simulink library "myo_lib"  (R2019b)
settings: Solver=ode45  StartTime=0.0  StopTime=10.0  RelTol=1e-3  EnableMultiTasking=on
settings Model: Creator=Mark Tomaszewski  LastModifiedBy=bhisma
settings DataIOCC: LimitDataPoints=on  SaveFormat=Array  ReturnWorkspaceOutputs=off
settings OptimizationCC: LifeSpan=inf
settings DebuggingCC: UnderspecifiedInitializationDetection=Classic  MergeDetectMultiDrivingBlocksExec=none  SolverPrmCheckMsg=warning  StateNameClashWarn=warning  SFUnexpectedBacktrackingDiag=warning  SFNoUnconditionalDefaultTransitionDiag=warning  SFExecutionAtInitializationDiag=none  ArithmeticOperatorsInVariantConditions=warning
settings HardwareCC: ProdBitPerPointer=32  ProdBitPerSizeT=32  ProdBitPerPtrDiffT=32  ProdLargestAtomicFloat=None  ProdIntDivRoundTo=Undefined  ProdEndianess=Unspecified  ProdWordSize=32  ProdHWDeviceType=32-bit Generic
settings ModelReferenceCC: PropagateSignalLabelsOutOfModel=off
settings SFSimCC: SimUseLocalCustomCode=off  CustomCodeUndefinedFunction=UseInterfaceOnly
settings RTWCC: RTWUseLocalCustomCode=off
settings CodeAppCC: StateflowObjectComments=on
settings GRTTargetCC: TargetLangStandard=C89/C90 (ANSI)  GeneratePreprocessorConditionals=Disable all
settings ConfigComp: CovMetricSettings=dw  CovHtmlReporting=on  CovSaveCumulativeToWorkspaceVar=on  CovSaveSingleToWorkspaceVar=on  CovExternalEMLEnable=off

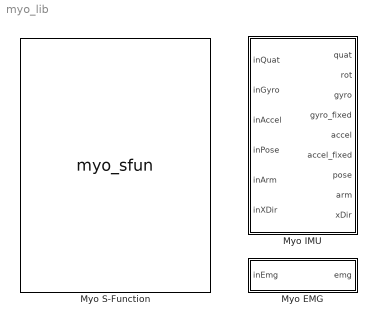
== system myo_lib ==
  Myo EMG : Subsystem
  Myo IMU : Subsystem
  Myo S-Function : S-Function  FunctionName=myo_sfun  Parameters=emgEnabled,countMyos  SFunctionDeploymentMode=off  EnableBusSupport=off  mask{emgEnabled=1, countMyos=1}
      mask prompts: emgEnabled "EMG Enabled (1 to set or 0 to unset)"; countMyos "Count Myos (1 or 2)"
      mask init:
      | disp init-mask
      mask Callback emgEnabled: myo_sfun_param_cb(gcb)
      mask Callback countMyos: myo_sfun_param_cb(gcb)
      mask Display:
      | %myo_sfun_draw_cb(gcb);
      | 
      | text(0.1,0.9,'Myo\nS-Function')
      | 
      | % default ports
      | port_label('output',1,'myoData(1).quat')
      | port_label('output',2,'myoData(1).gyro')
      | port_label('output',3,'myoData(1).accel')
      | port_label('output',4,'myoData(1).pose')
      | port_label('output',5,'myoData(1).arm')
      | port_label('output',6,'myoData(1).xDir')
      | 
      | % emg
      | if emgEnabled==1
      |   port_label('output',7,'myoData(1).emg')
      | end
      | 
      | % myo2
      | if countMyos==2
      |   port_label('output',7,'myoData(2).quat')
      |   port_label('output',8,'myoData(2).gyro')
      |   port_label('output',9,'myoData(2).accel')
      |   port_label('output',10,'myoData(2).pose')
      |   port_label('output',11,'myoData(2).arm')
      |   port_label('output',12,'myoData(2).xDir')
      | end

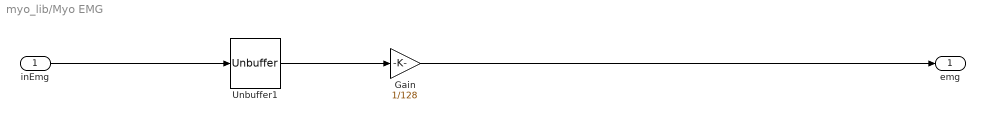
== system myo_lib/Myo EMG ==
  inEmg : Inport
  Gain : Gain  Gain=1/128
  Unbuffer1 : Unbuffer
  emg : Outport
  wires:
  Unbuffer1/1 -> Gain/1
  inEmg/1 -> Unbuffer1/1
  Gain/1 -> emg/1

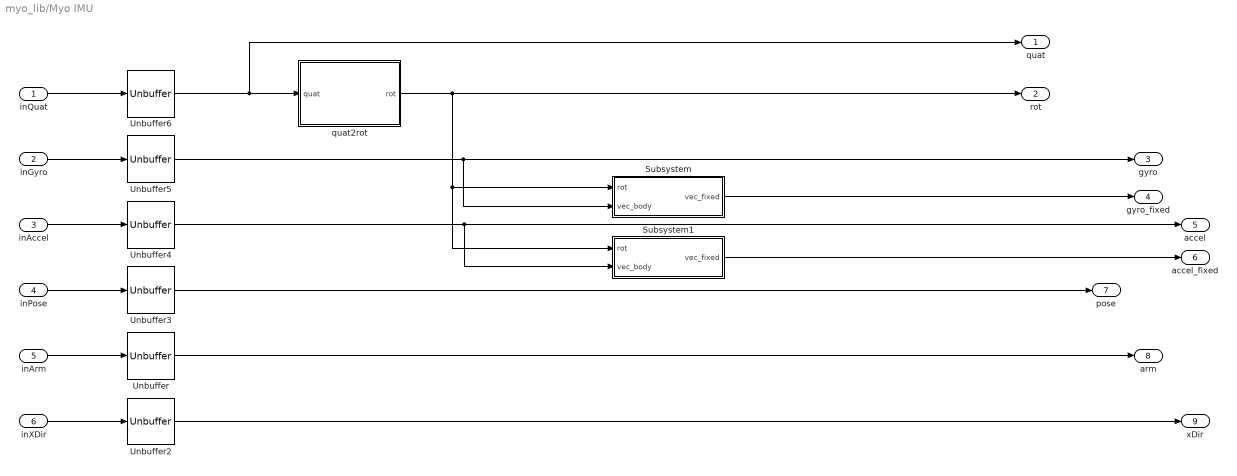
== system myo_lib/Myo IMU ==
  inQuat : Inport
  inGyro : Inport  Port=2
  inAccel : Inport  Port=3
  inPose : Inport  Port=4
  inArm : Inport  Port=5
  inXDir : Inport  Port=6
  Subsystem : Subsystem
  Subsystem1 : Subsystem
  Unbuffer{,2..5} (5 alike) : Unbuffer
  Unbuffer6 : Unbuffer  ic=[1,0,0,0;1,0,0,0]
  quat2rot : Subsystem
  quat : Outport
  rot : Outport  Port=2
  gyro : Outport  Port=3
  gyro_fixed : Outport  Port=4
  accel : Outport  Port=5
  accel_fixed : Outport  Port=6
  pose : Outport  Port=7
  arm : Outport  Port=8
  xDir : Outport  Port=9
  wires:
  Unbuffer3/1 -> pose/1
  inGyro/1 -> Unbuffer5/1
  Unbuffer6/1 -> quat/1, quat2rot/1(quat)
  Unbuffer4/1 -> Subsystem1/2(vec_body), accel/1
  Unbuffer5/1 -> Subsystem/2(vec_body), gyro/1
  inPose/1 -> Unbuffer3/1
  inArm/1 -> Unbuffer/1
  inAccel/1 -> Unbuffer4/1
  Unbuffer/1 -> arm/1
  inXDir/1 -> Unbuffer2/1
  inQuat/1 -> Unbuffer6/1
  Unbuffer2/1 -> xDir/1
  quat2rot/1(rot) -> rot/1, Subsystem1/1(rot), Subsystem/1(rot)
  Subsystem/1(vec_fixed) -> gyro_fixed/1
  Subsystem1/1(vec_fixed) -> accel_fixed/1

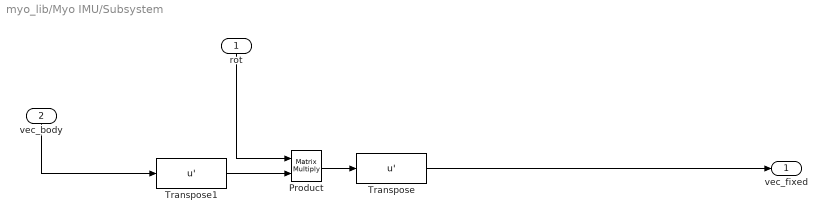
== system myo_lib/Myo IMU/Subsystem ==
  rot : Inport
  vec_body : Inport  Port=2
  Product : Product  Multiplication=Matrix(*)
  Transpose : MATLABFcn  MATLABFcn=u'  Output1D=off
  Transpose1 : MATLABFcn  MATLABFcn=u'  Output1D=off
  vec_fixed : Outport
  wires:
  Product/1 -> Transpose/1
  Transpose1/1 -> Product/2
  vec_body/1 -> Transpose1/1
  rot/1 -> Product/1
  Transpose/1 -> vec_fixed/1

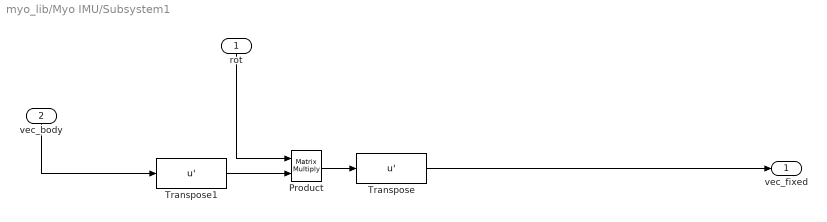
== system myo_lib/Myo IMU/Subsystem1 ==
  rot : Inport
  vec_body : Inport  Port=2
  Product : Product  Multiplication=Matrix(*)
  Transpose : MATLABFcn  MATLABFcn=u'  Output1D=off
  Transpose1 : MATLABFcn  MATLABFcn=u'  Output1D=off
  vec_fixed : Outport
  wires:
  Product/1 -> Transpose/1
  Transpose1/1 -> Product/2
  vec_body/1 -> Transpose1/1
  rot/1 -> Product/1
  Transpose/1 -> vec_fixed/1

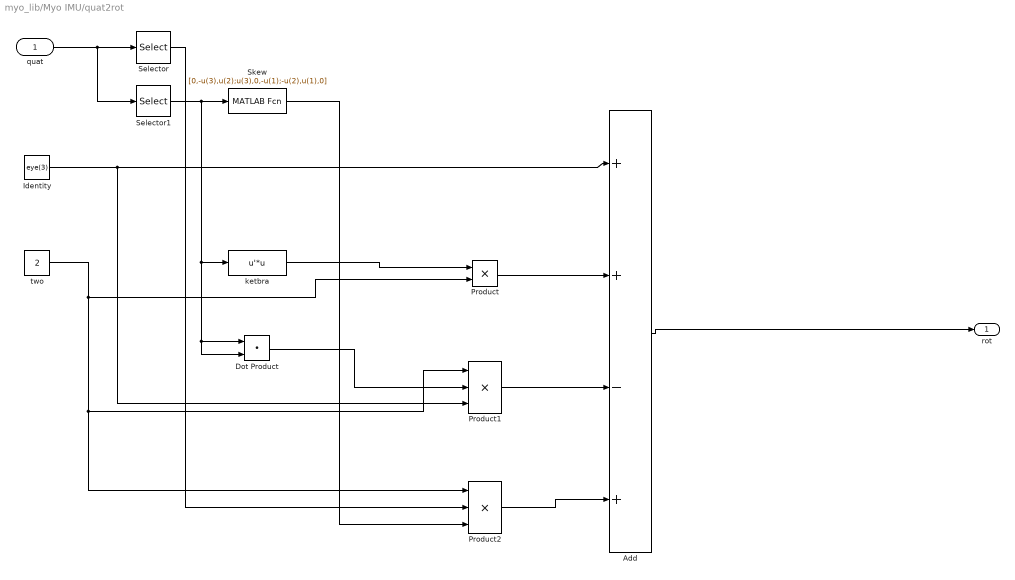
== system myo_lib/Myo IMU/quat2rot ==
  quat : Inport
  Add : Sum  Inputs=++-+
  Dot Product : DotProduct  InputSameDT=on  OutDataTypeStr=Inherit: Inherit via internal rule
  Identity : Constant  Value=eye(3)
  Product : Product
  Product1 : Product  Inputs=3
  Product2 : Product  Inputs=3
  Selector : Selector  InputPortWidth=4  IndexOptions=Index vector (dialog)  Indices=[1]  OutputSizes=1
  Selector1 : Selector  InputPortWidth=4  IndexOptions=Index vector (dialog)  Indices=[2,3,4]  OutputSizes=1
  Skew : MATLABFcn  MATLABFcn=[0,-u(3),u(2);u(3),0,-u(1);-u(2),u(1),0]  Output1D=off
  ketbra : MATLABFcn  MATLABFcn=u'*u  Output1D=off
  two : Constant  Value=2
  rot : Outport
  wires:
  quat/1 -> Selector/1, Selector1/1
  Selector1/1 -> Dot Product/2, Dot Product/1, ketbra/1, Skew/1
  Add/1 -> rot/1
  Identity/1 -> Product1/3, Add/1
  Skew/1 -> Product2/3
  ketbra/1 -> Product/1
  Product/1 -> Add/2
  two/1 -> Product2/1, Product1/1, Product/2
  Dot Product/1 -> Product1/2
  Product1/1 -> Add/3
  Selector/1 -> Product2/2
  Product2/1 -> Add/4
